simulink model "LWR4"  (R2016b)
settings: Solver=FixedStepDiscrete  StartTime=0  StopTime=4  FixedStep=0.1  MaxStep=0.010  RelTol=1e-3  EnableMultiTasking=on
InitFcn:
  | clear all
  | clc
  | 
  | global clientID
  | global vrep
  | global vecJoints nJoints
  | 
  | load_path
  | 
  | 
  | addpath('C:\Program Files\V-REP3\V-REP_PRO_EDU\programming\remoteApiBindings\lib\lib\Windows\64Bit')
  | 
  | 
  | disp('Program started');
  | vrep=remApi('remoteApi'); % using the prototype file (remoteApiProto.m)
  | vrep.simxFinish(-1); % just in case, close all opened connections
  | clientID=vrep.simxStart('127.0.0.1',19997,true,true,5000,5);
  | 
  | vrep.simxStartSimulation(clientID,vrep.simx_opmode_oneshot_wait);
  | vrep.simxSynchronous(clientID,true)
  | 
  | if (clientID<=-1)
  |     disp('stop simulation')
  |     vrep.delete();
  |     set_param(gcs, 'SimulationCommand', 'stop')
  | end
  | 
  | % Root of the joint in Vrep
  | rootJoints     = 'UR10_joint';
  | 
  | % Number of joints
  | nJoints        = 6;
  | 
  | % Handles of the joints
  | vecJoints      = zeros(nJoints,1);
  | 
  | for i=1:nJoints
  |                 [res,obj]=vrep.simxGetObjectHandle(clientID,strcat(rootJoints,int2str(i)),vrep.simx_opmode_oneshot_wait);
  |                 if res==vrep.simx_return_ok
  |                     vecJoints(i) = obj;
  |                    [res,pos] = vrep.simxGetJointPosition(clientID,vecJoints(i),vrep.simx_opmode_streaming);
  |                 else
  |                     vecJoints(i) = -1;
  |                     disp(strcat('joint nr ', int2str(i), ' named ', rootJoints, int2str(i) , ' not avalaible!'));
  |                 end
  | end
StopFcn:
  | global clientID
  | 
  | vrep.simxStopSimulation(clientID,vrep.simx_opmode_oneshot_wait);
settings Model: Creator=Massimo  LastModifiedBy=IBM
settings DataIOCC: LimitDataPoints=on  SaveFormat=Array
settings OptimizationCC: LifeSpan=inf
settings DebuggingCC: UnderspecifiedInitializationDetection=Classic  MergeDetectMultiDrivingBlocksExec=none  StateNameClashWarn=warning  SFUnexpectedBacktrackingDiag=warning  SFNoUnconditionalDefaultTransitionDiag=warning  SFExecutionAtInitializationDiag=none
settings HardwareCC: ProdBitPerPointer=32  ProdBitPerSizeT=32  ProdBitPerPtrDiffT=32  ProdLargestAtomicFloat=None  ProdIntDivRoundTo=Undefined  ProdEndianess=Unspecified  ProdWordSize=32  ProdHWDeviceType=32-bit Generic
settings ModelReferenceCC: PropagateSignalLabelsOutOfModel=off
settings GRTTargetCC: TargetLangStandard=C89/C90 (ANSI)  GeneratePreprocessorConditionals=Disable all
settings ConfigComp: CovMetricSettings=dw  CovHtmlReporting=on  CovSaveCumulativeToWorkspaceVar=on  CovSaveSingleToWorkspaceVar=on  CovExternalEMLEnable=off

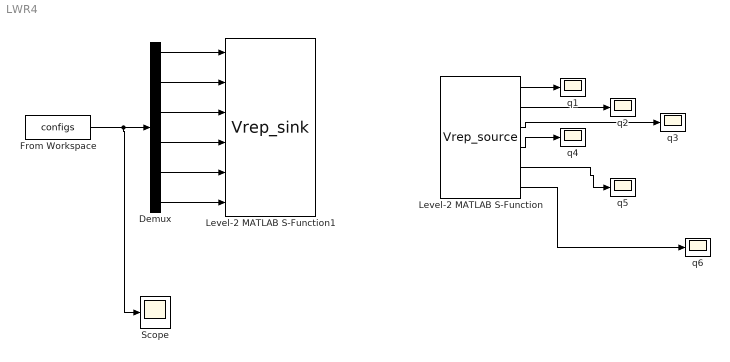
== system LWR4 ==
  Demux : Demux  Outputs=6
  From Workspace : FromWorkspace  VariableName=configs  OutDataTypeStr=double  SampleTime=0
  Level-2 MATLAB S-Function : M-S-Function  FunctionName=Vrep_source
  Level-2 MATLAB S-Function1 : M-S-Function  FunctionName=Vrep_sink
  Scope : Scope
  q{1..6} (6 alike) : Scope
  wires:
  Level-2 MATLAB S-Function/1 -> q1/1
  Level-2 MATLAB S-Function/2 -> q2/1
  Level-2 MATLAB S-Function/3 -> q3/1
  Level-2 MATLAB S-Function/4 -> q4/1
  Level-2 MATLAB S-Function/5 -> q5/1
  Level-2 MATLAB S-Function/6 -> q6/1
  Demux/4 -> Level-2 MATLAB S-Function1/4
  Demux/5 -> Level-2 MATLAB S-Function1/5
  Demux/3 -> Level-2 MATLAB S-Function1/3
  Demux/2 -> Level-2 MATLAB S-Function1/2
  Demux/1 -> Level-2 MATLAB S-Function1/1
  Demux/6 -> Level-2 MATLAB S-Function1/6
  From Workspace/1 -> Scope/1, Demux/1
